simulink model "DigitalTwin"  (R2023b)
settings: Solver=ode23t  StartTime=0.0  StopTime=600  RelTol=1e-3  AbsTol=1e-3
model workspace: external: MATLAB File C:\Users\claud\OneDrive - TUM\COME -TUM\Software lab\Three_wheeled_base\simscape_1\Three_wheeled_base_DataFile1.m (data not in the file)
values from neighbouring files (symbols this model uses):
  brick_pick_global_xy = [brick_pick_global_xy, new_column]    [Three_wheeled_base_LOAD_DATA.m]
  brick_place_global_xy = [brick_place_global_xy, new_column]    [Three_wheeled_base_LOAD_DATA.m]
  platform_destination_mat = [ 1.0 0; 5 0; 0 0; 0 5 ... (first row only)    [Three_wheeled_base_LOAD_DATA.m]
undefined symbols (not defined in the file or in its folder): robotData, smiData, X, Y, Z
libraries: sm_lib x237, nesl_utility x78, fl_lib x12, batteryecm_lib x5, ee_lib x3, robotcorelib x1, robotalgslib x1
(part 1 of 7)
settings Model: Creator=claud  LastModifiedBy=Claudia
settings SolverCC: AutoScaleAbsTol=off
settings SFSimCC: LegacyBehaviorForPersistentVarInContinuousTime=on
settings SimscapeCC: SimscapeLogType=all
settings ExplorerConfigSet: InternalSimMechanicsExplorerSettings="<ExplorerConfiguration><canonicalview>default</canonicalview><AnimationSetting><BasePlaybackSpeed>1.0</BasePlaybackSpeed><PlaybackSpeedFactor>1.0</PlaybackSpeedFactor></AnimationSetting><TilePanel><TileInfo><Tiles Columns=\"1\" Count=\"1\" Rows=\"1\"><Column Weight=\"1\"/><Row Weight=\"1\"/><Tile Height=\"1\" Width=\"1\" X=\"0\" Y=\"0\"/></Tiles></TileInfo><SceneInfo><SceneViewer><BGColor><R>0.60000002384185791</R><G>0.60000002384185791</G><B>0.60000002384185791</B></BGColor><Camera><DoPerspective>on</DoPerspective><Position><X>1.00584110741406163</X><Y>1.01006722214987787</Y><Z>1.41600001786290575</Z></Position><Center><X>0.00584110741406168588</X><Y>0.0100672221498779302</Y><Z>0.416000017862905691</Z></Center><Up><X>0</X><Y>1</Y><Z>0</Z></Up><ViewLimDist>1</ViewLimDist><YLim>0.466307658154998583</YLim><XLim>0.724334873452957884</XLim></Camera></SceneViewer></SceneInfo></TilePanel><MechEditorPanel><Cameras><Camera><Id>Camera1</Id><Value><Name>iso_FR</Name><NativeCamera><PositionTrackingFeature>Cam.F</PositionTrackingFeature><CenterTrackingFeature>Base_1_RIGID.Solid.R</CenterTrackingFeature><UpVectorTrackingFeature>World.W</UpVectorTrackingFeature><CenterTrackingOrigin>on</CenterTrackingOrigin><UpVectorTrackingDirection>+Y</UpVectorTrackingDirection></NativeCamera></Value></Camera></Cameras><GfxPanelCameraMap><MapElement CameraMLId=\"Camera1\" GfxPanelIndex=\"0\"/></GfxPanelCameraMap><VideoCreator><PlaybackSpeedRatio>1.0</PlaybackSpeedRatio><FrameRate>30</FrameRate><VideoFormat>Motion JPEG AVI</VideoFormat><FrameSize>auto</FrameSize></VideoCreator></MechEditorPanel></ExplorerConfiguration>"

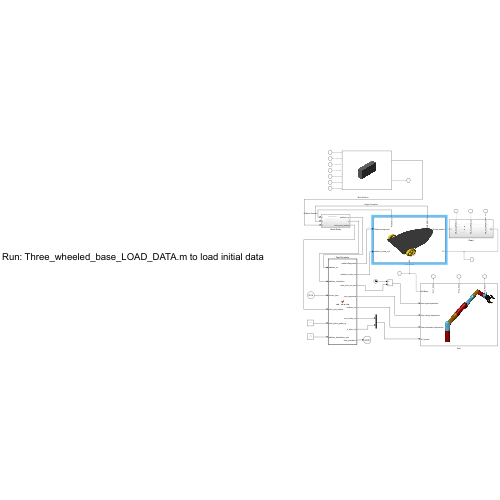
[thumbnail: Simulink's stored preview of the top-level diagram]
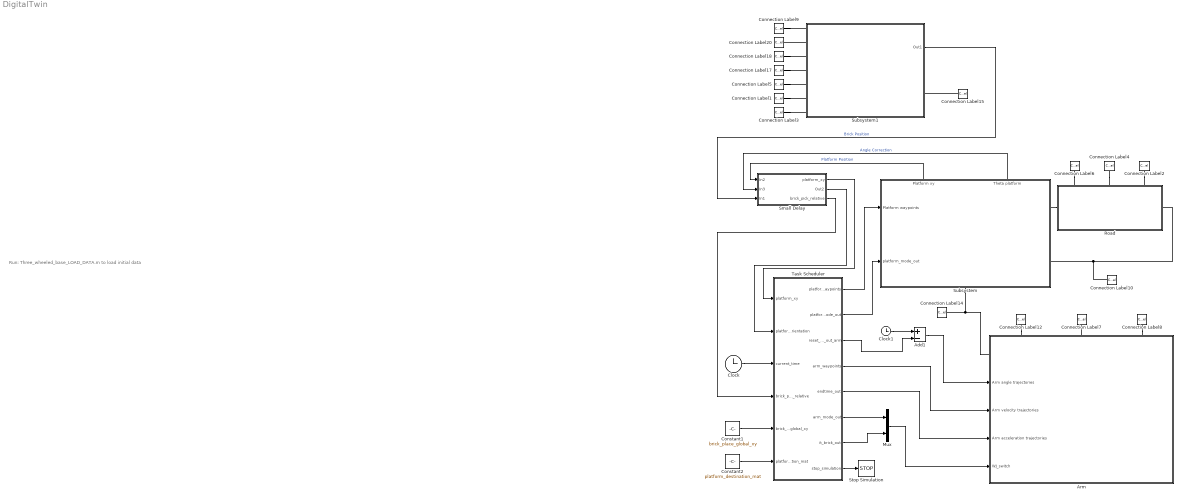
== system DigitalTwin ==
  note: Run: Three_wheeled_base_LOAD_DATA.m to load initial data
  Add1 : Sum  Inputs=+-
  Arm : Subsystem
      settings: PortSchema="{\"entries\":[{\"content\":{\"sides\":[{\"content\":{\"connectorIds\":[\"LConn1\",\"In1\",\"In2\",\"In3\",\"In4\"]},\"type\":\"ConnectorPlacement.EquallySpacedRectSide\",\"uuid\":\"ee2274a6-58ed-4bc3-bc3c-ce92a4d8f88b\"},{\"content\":{\"side\":\"RIGHT\"},\"type\":\"ConnectorPlacement.EquallySpacedRectSide\",\"uuid\":\"7a54403a-43fc-49b7-a0b4-bb229ee477d3\"},{\"content\":{\"connectorIds\":[\"LConn2\",\"LConn3\",\"LConn4\"],\"side\":\"TOP\"},\"type\":\"ConnectorPlacement.EquallySpacedRectSide\",\"uuid\":\"23c7f7d7-6525-440f-a2bd-2c7519a630a0\"}]},\"type\":\"ConnectorPlacement.EquallySpacedConnector\",\"uuid\":\"ecb498cc-d8ef-4f5d-a849-59a03134dc5f\"}],\"packageUris\":[\"http://schema.mathworks.com/mf0/Connector/R2020b\"],\"version\":\"1.0\"}"
      mask Display: image('arm.png');
  Clock : Clock
  Clock1 : Clock
  Connection Label1 : ConnectionLabel  Label=WJ2
  Connection Label10 : ConnectionLabel  Label=World_Ref
  Connection Label12 : ConnectionLabel  Label=WJ1
  Connection Label14 : ConnectionLabel  Label=Base_Ref
  Connection Label15 : ConnectionLabel  Label=Base_Ref
  Connection Label17 : ConnectionLabel  Label=BG_Contact3
  Connection Label18 : ConnectionLabel  Label=BG_Contact2
  Connection Label2 : ConnectionLabel  Label=BG_Contact3
  Connection Label20 : ConnectionLabel  Label=BG_Contact1
  Connection Label3 : ConnectionLabel  Label=WJ3
  Connection Label4 : ConnectionLabel  Label=BG_Contact2
  Connection Label5 : ConnectionLabel  Label=WJ1
  Connection Label6 : ConnectionLabel  Label=BG_Contact1
  Connection Label7 : ConnectionLabel  Label=WJ2
  Connection Label8 : ConnectionLabel  Label=WJ3
  Connection Label9 : ConnectionLabel  Label=World_Ref
  Constant1 : Constant  Value=brick_place_global_xy
  Constant2 : Constant  Value=platform_destination_mat
  Mux : Mux  Inputs=2
  Road : Subsystem
      settings: PortSchema="{\"entries\":[{\"content\":{\"sides\":[{\"content\":{\"connectorIds\":[\"LConn1\"]},\"type\":\"ConnectorPlacement.EquallySpacedRectSide\",\"uuid\":\"262a7389-5f19-4e57-b137-adc0fe64cf6a\"},{\"content\":{\"connectorIds\":[\"RConn1\"],\"side\":\"RIGHT\"},\"type\":\"ConnectorPlacement.EquallySpacedRectSide\",\"uuid\":\"0021701d-9431-401f-ab56-f5ab9263888d\"},{\"content\":{\"connectorIds\":[\"LConn2\",\"LConn3\",\"LConn4\"],\"side\":\"TOP\"},\"type\":\"ConnectorPlacement.EquallySpacedRectSide\",\"uuid\":\"4d80399b-ee48-44ac-89eb-a0f63eadeb61\"}]},\"type\":\"ConnectorPlacement.EquallySpacedConnector\",\"uuid\":\"517c2f99-1dab-4bb3-8d67-634ce2b33fa0\"}],\"packageUris\":[\"http://schema.mathworks.com/mf0/Connector/R2020b\"],\"version\":\"1.0\"}"
  Small Delay : Subsystem
  Stop Simulation : Stop
  Subsystem : Subsystem
      settings: PortSchema="{\"entries\":[{\"content\":{\"sides\":[{\"content\":{\"connectorIds\":[\"In1\",\"In2\"]},\"type\":\"ConnectorPlacement.EquallySpacedRectSide\",\"uuid\":\"4ac1efda-dcc9-454e-8ad9-ce8f4f6e0b89\"},{\"content\":{\"connectorIds\":[\"RConn1\",\"RConn2\"],\"side\":\"RIGHT\"},\"type\":\"ConnectorPlacement.EquallySpacedRectSide\",\"uuid\":\"c7ac7953-1964-411a-9b01-00f16356f779\"},{\"content\":{\"connectorIds\":[\"Out1\",\"Out2\"],\"side\":\"TOP\"},\"type\":\"ConnectorPlacement.EquallySpacedRectSide\",\"uuid\":\"7737e004-77be-4cf9-a6ff-a2bb3522befd\"},{\"content\":{\"connectorIds\":[\"RConn3\"],\"side\":\"BOTTOM\"},\"type\":\"ConnectorPlacement.EquallySpacedRectSide\",\"uuid\":\"51c42121-fb18-4794-8883-c90eb5d184da\"}]},\"type\":\"ConnectorPlacement.EquallySpacedConnector\",\"uuid\":\"70e365d4-4171-4d10-b657-56f628ea464d\"}],\"packageUris\":[\"http://schema.mathworks.com/mf0/Connector/R2020b\"],\"version\":\"1.0\"}"
      mask Display: image('platform.png');
  Subsystem1 : Subsystem
      mask Display: image('brick.png'); % Use "Edit Image" on toolstrip to change.
  Task Scheduler : MATLAB Function  TreatAsAtomicUnit=on
  wires:
  Mux/1 -> Arm/4(WJ_switch)
  Constant2/1 -> Task Scheduler/6(platform_destination_mat)
  Task Scheduler/5(endtime_out) -> Arm/3(Arm acceleration trajectories)
  Task Scheduler/1(platformWaypoints) -> Subsystem/1(Platform waypoints)
  Task Scheduler/7(it_brick_out) -> Mux/2
  Task Scheduler/2(platform_mode_out) -> Subsystem/2(platform_mode_out)
  Clock1/1 -> Add1/1
  Constant1/1 -> Task Scheduler/5(brick_place_global_xy)
  Task Scheduler/3(reset_time_out_arm) -> Add1/2
  Task Scheduler/4(arm_waypoints) -> Arm/2(Arm velocity trajectories)
  Clock/1 -> Task Scheduler/3(current_time)
  Task Scheduler/6(arm_mode_out) -> Mux/1
  Add1/1 -> Arm/1(Arm angle trajectories)
  Task Scheduler/8(stop_simulation) -> Stop Simulation/1
  Subsystem1/1(Out1) -> Small Delay/3(In1)  "Brick Position"
  Subsystem/1(Platform xy) -> Small Delay/1(In2)  "Platform Position"
  Subsystem/2(Theta platform) -> Small Delay/2(In3)  "Angle Correction"
  Small Delay/1(platform_xy) -> Task Scheduler/1(platform_xy)
  Small Delay/2(Out2) -> Task Scheduler/2(platform_orientation)
  Small Delay/3(brick_pick_relative) -> Task Scheduler/4(brick_pick_relative)
  connections:
  Subsystem/RConn1 -- Road/LConn1
  Connection Label9/LConn1 -- Subsystem1/LConn1
  Connection Label18/LConn1 -- Subsystem1/LConn3
  Subsystem/RConn3 -- Arm/LConn1 -- Connection Label14/LConn1
  Connection Label3/LConn1 -- Subsystem1/LConn7
  Connection Label15/LConn1 -- Subsystem1/RConn1
  Connection Label17/LConn1 -- Subsystem1/LConn4
  Connection Label1/LConn1 -- Subsystem1/LConn6
  Connection Label5/LConn1 -- Subsystem1/LConn5
  Subsystem1/LConn2 -- Connection Label20/LConn1
  Connection Label2/LConn1 -- Road/LConn4
  Connection Label4/LConn1 -- Road/LConn3
  Connection Label6/LConn1 -- Road/LConn2
  Connection Label10/LConn1 -- Subsystem/RConn2 -- Road/RConn1
  Arm/LConn3 -- Connection Label7/LConn1
  Connection Label8/LConn1 -- Arm/LConn4
  Connection Label12/LConn1 -- Arm/LConn2

== system DigitalTwin/Arm ==
  Arm angle trajectories : Inport
  Arm velocity trajectories : Inport  Port=2
  Arm acceleration trajectories : Inport  Port=3
  WJ_switch : Inport  Port=4
  Kinova Gen3 Arm : Subsystem
      settings: PortSchema="{\"entries\":[{\"content\":{\"sides\":[{\"content\":{\"connectorIds\":[\"In1\",\"In2\",\"In3\",\"In4\",\"LConn1\"]},\"type\":\"ConnectorPlacement.EquallySpacedRectSide\",\"uuid\":\"9d5091ef-fb90-4975-9d40-26cfdfa951d0\"},{\"content\":{\"side\":\"RIGHT\"},\"type\":\"ConnectorPlacement.EquallySpacedRectSide\",\"uuid\":\"b105551f-355d-4434-964a-24d22199b3bd\"},{\"content\":{\"side\":\"TOP\"},\"type\":\"ConnectorPlacement.EquallySpacedRectSide\",\"uuid\":\"70b9d2f5-4ba7-485a-93bc-ea7c6d2c4586\"},{\"content\":{\"connectorIds\":[\"RConn1\",\"RConn2\",\"RConn3\"],\"side\":\"BOTTOM\"},\"type\":\"ConnectorPlacement.EquallySpacedRectSide\",\"uuid\":\"265168f2-3491-4ded-adb5-35e09b8a8943\"}]},\"type\":\"ConnectorPlacement.EquallySpacedConnector\",\"uuid\":\"3d8cb1a4-1099-498e-9732-6de55f59cc0e\"}],\"packageUris\":[\"http://schema.mathworks.com/mf0/Connector/R2020b\"],\"version\":\"1.0\"}"
  Trapezoidal Velocity Profile Trajectory Robotic arm : robotcorelib/Trapezoidal Velocity Profile Trajectory  WaypointSource=External  Waypoints=waypoints  NumParams=1  Parameter1=End Time  Parameter2=End Time  ParameterSource=External  PeakVelocity=[ 2; 2 ]  Acceleration=[ 1; 2 ]  EndTime=10  AccelTime=[ 1; 2 ]  SimulateUsing=Interpreted execution
  Ref Base : PMIOPort  Side=Left
  WJ1_Fport : PMIOPort  Port=2  Side=Left
  WJ2_Fport : PMIOPort  Port=3  Side=Left
  WJ2_Fport1 : PMIOPort  Port=4  Side=Left
  wires:
  WJ_switch/1 -> Kinova Gen3 Arm/4(WJ_switch)
  Arm angle trajectories/1 -> Trapezoidal Velocity Profile Trajectory Robotic arm/1
  Arm velocity trajectories/1 -> Trapezoidal Velocity Profile Trajectory Robotic arm/2
  Arm acceleration trajectories/1 -> Trapezoidal Velocity Profile Trajectory Robotic arm/3
  Trapezoidal Velocity Profile Trajectory Robotic arm/1 -> Kinova Gen3 Arm/1(Angle)
  Trapezoidal Velocity Profile Trajectory Robotic arm/2 -> Kinova Gen3 Arm/2(Velocity)
  Trapezoidal Velocity Profile Trajectory Robotic arm/3 -> Kinova Gen3 Arm/3(Acceleration)
  connections:
  WJ1_Fport/RConn1 -- Kinova Gen3 Arm/RConn1
  Ref Base/RConn1 -- Kinova Gen3 Arm/LConn1
  Kinova Gen3 Arm/RConn2 -- WJ2_Fport/RConn1
  WJ2_Fport1/RConn1 -- Kinova Gen3 Arm/RConn3

== system DigitalTwin/Road ==
  Infinite Plane : sm_lib/Curves and Surfaces/Infinite Plane  GraphicType=None  GraphicPlaneWidth=20  GraphicPlaneWidthUnits=m  GraphicPlaneHeight=20  GraphicPlaneHeightUnits=m  GraphicVisPropType=SimpleVisualProperties  GraphicDiffuseColor=[0.5 0.5 0.5]  GraphicOpacity=0.25  GraphicSpecularColor=[0.5 0.5 0.5 1.0]  GraphicAmbientColor=[0.15 0.15 0.15 1.0]  GraphicEmissiveColor=[0.0 0.0 0.0 1.0]  GraphicShininess=75
  Infinite Transform : sm_lib/Frames and Transforms/Rigid Transform  TranslationMethod=Cartesian  TranslationStandardOffset=0  TranslationStandardOffsetUnits=m  TranslationStandardAxis=+Z  TranslationCartesianOffset=[-1 -0.1 0]  TranslationCartesianOffsetUnits=m  TranslationROffset=0  TranslationROffsetUnits=m  TranslationZOffset=0  TranslationZOffsetUnits=m  TranslationThetaOffset=0  TranslationThetaOffsetUnits=deg  RotationMethod=StandardAxis  RotationAngleUnits=deg  RotationStandardAxis=-X  RotationAngle=0.0  RotationArbitraryAxis=[0 0 1]  FollAlignAxisA=+X  BaseAlignAxisA=+Y  FollAlignAxisB=+Y  BaseAlignAxisB=+Z  RotationSequenceAxes=FollowerAxes  RotationSequence=XYX  RotationSequenceAngles=[0 0 0]  RotationSequenceAnglesUnits=deg  RotationMatrix=[1 0 0; 0 1 0; 0 0 1]  Quaternion=[1 0 0 0]
  Spatial Contact Force : sm_lib/Forces and Torques/Spatial Contact Force  SenseContactBaseRotation=off  SenseContactBaseTranslation=off  CoefficientOfDynamicFriction=0.3  CoefficientOfStaticFriction=0.5  NormalDamping=1e3  NormalDampingUnits=N/(m/s)  SenseContactSignal=off  NormalStiffness=1e6  NormalStiffnessUnits=N/m  FrictionalCriticalVelocity=1e-3  FrictionalCriticalVelocityUnits=m/s  ZeroCrossDetectContactStartAndEnd=off  SenseContactFollowerRotation=off  SenseContactFollowerTranslation=off  FrictionType=SmoothStickSlip  SenseFrictionalForceMagnitude=off  SenseNormalForceMagnitude=off  NormalForceType=SmoothSpringDamper  SenseNormalVelocity=off  SensePenetrationDepth=off  SenseSeparationDistance=off  SenseTangentialVelocity=off  NormalTransitionRegionWidth=1e-4  NormalTransitionRegionWidthUnits=m
  Spatial Contact Force1 : sm_lib/Forces and Torques/Spatial Contact Force  SenseContactBaseRotation=off  SenseContactBaseTranslation=off  CoefficientOfDynamicFriction=0.3  CoefficientOfStaticFriction=0.5  NormalDamping=1e3  NormalDampingUnits=N/(m/s)  SenseContactSignal=off  NormalStiffness=1e6  NormalStiffnessUnits=N/m  FrictionalCriticalVelocity=1e-3  FrictionalCriticalVelocityUnits=m/s  ZeroCrossDetectContactStartAndEnd=off  SenseContactFollowerRotation=off  SenseContactFollowerTranslation=off  FrictionType=SmoothStickSlip  SenseFrictionalForceMagnitude=off  SenseNormalForceMagnitude=off  NormalForceType=SmoothSpringDamper  SenseNormalVelocity=off  SensePenetrationDepth=off  SenseSeparationDistance=off  SenseTangentialVelocity=off  NormalTransitionRegionWidth=1e-4  NormalTransitionRegionWidthUnits=m
  Spatial Contact Force2 : sm_lib/Forces and Torques/Spatial Contact Force  SenseContactBaseRotation=off  SenseContactBaseTranslation=off  CoefficientOfDynamicFriction=0.3  CoefficientOfStaticFriction=0.5  NormalDamping=1e3  NormalDampingUnits=N/(m/s)  SenseContactSignal=off  NormalStiffness=1e6  NormalStiffnessUnits=N/m  FrictionalCriticalVelocity=1e-3  FrictionalCriticalVelocityUnits=m/s  ZeroCrossDetectContactStartAndEnd=off  SenseContactFollowerRotation=off  SenseContactFollowerTranslation=off  FrictionType=SmoothStickSlip  SenseFrictionalForceMagnitude=off  SenseNormalForceMagnitude=off  NormalForceType=SmoothSpringDamper  SenseNormalVelocity=off  SensePenetrationDepth=off  SenseSeparationDistance=off  SenseTangentialVelocity=off  NormalTransitionRegionWidth=1e-4  NormalTransitionRegionWidthUnits=m
  F1 : PMIOPort  Side=Left
  F2 : PMIOPort  Port=2  Side=Right
  CF_CloudPoints1 : PMIOPort  Port=3  Side=Left
  CF_CloudPoints2 : PMIOPort  Port=4  Side=Left
  CF_CloudPoints3 : PMIOPort  Port=5  Side=Left
  connections:
  Infinite Transform/LConn1 -- F2/RConn1
  Infinite Plane/RConn1 -- Spatial Contact Force2/LConn1 -- Spatial Contact Force1/LConn1 -- Spatial Contact Force/LConn1 -- F1/RConn1
  Infinite Plane/LConn1 -- Infinite Transform/RConn1
  Spatial Contact Force/RConn1 -- CF_CloudPoints1/RConn1
  Spatial Contact Force1/RConn1 -- CF_CloudPoints2/RConn1
  Spatial Contact Force2/RConn1 -- CF_CloudPoints3/RConn1

== system DigitalTwin/Small Delay ==
  note: Continuous small delay
  In2 : Inport
  In3 : Inport  Port=2
  In1 : Inport  Port=3
  Reshape1 : Reshape  OutputDimensionality=Customize  OutputDimensions=9
  Reshape2 : Reshape  OutputDimensionality=Customize  OutputDimensions=[3,3]
  Small delay : Subsystem
  Small delay1 : Subsystem
  Transfer Fcn3 : TransferFcn  Denominator=[10^(-6) 1]
  platform_xy : Outport
  Out2 : Outport  Port=2
  brick_pick_relative : Outport  Port=3
  wires:
  In1/1 -> Reshape1/1
  Small delay/1(Out1) -> Reshape2/1
  In3/1 -> Transfer Fcn3/1
  Reshape1/1 -> Small delay/1(In1)
  Transfer Fcn3/1 -> Out2/1
  Small delay1/1(platform_xy) -> platform_xy/1
  Reshape2/1 -> brick_pick_relative/1
  In2/1 -> Small delay1/1(In1)
